simulink model "test_road"  (Simulink 7.6)
settings: Solver=ode3  StartTime=0.0  StopTime=10  FixedStep=.05  RelTol=1e-3
PostLoadFcn:
  | Threshold = 15;
  | MaxCluster = 25;
  | Num_Beams = 726;
  | Scaling = 1;
  | javaaddpath({'/'});
  | import ClusterMethodRoad.*;
  | DataCluster = ClusterMethodRoad(Threshold,MaxCluster,Scaling,8,0.33);
  | eml.extrinsic('evalin');
StartFcn:
  | md_scan(0);
StopFcn:
  | md_scan(2);
libraries: realtime_pacer_lib x1
settings Model: Creator=TCA  LastModifiedBy=Elliot
settings OptimizationCC: InitFltsAndDblsToZero=on
settings DebuggingCC: StrictBusMsg=Warning
settings SFSimCC: SimParseCustomCode=off

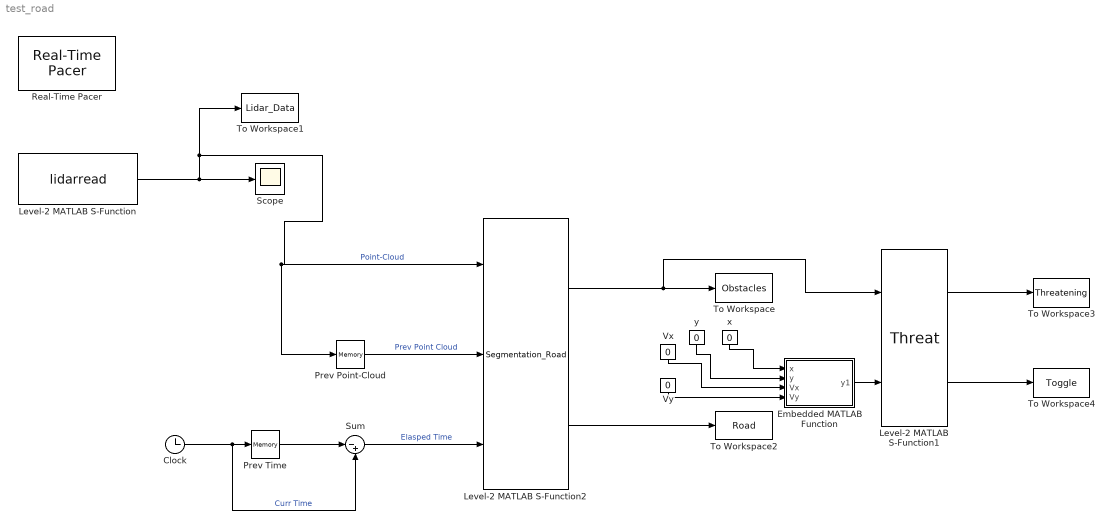
== system test_road ==
  Clock : Clock
      settings: Decimation=10
  Embedded MATLAB Function : Stateflow chart  TreatAsAtomicUnit=on
  Level-2 MATLAB S-Function : M-S-Function  FunctionName=lidarread
  Level-2 MATLAB S-Function1 : M-S-Function  FunctionName=Threat  Parameters=0.5,14,0.5
  Level-2 MATLAB S-Function2 : M-S-Function  FunctionName=Segmentation_Road
  Prev Point-Cloud : Memory
  Prev Time : Memory
  Real-Time Pacer : realtime_pacer_lib/Real-Time Pacer  simTimePerRealTime=1
  Scope : Scope
  Sum : Sum  Inputs=|-+
  To Workspace : ToWorkspace  VariableName=Obstacles  SampleTime=-1  SaveFormat=Structure
  To Workspace1 : ToWorkspace  VariableName=Lidar_Data  SampleTime=-1  SaveFormat=Structure With Time
  To Workspace2 : ToWorkspace  VariableName=Road  SampleTime=-1  SaveFormat=Structure
  To Workspace3 : ToWorkspace  VariableName=Threatening  SampleTime=-1  SaveFormat=Structure
  To Workspace4 : ToWorkspace  VariableName=Toggle  SampleTime=-1  SaveFormat=Array
  Vx : Constant  Value=0
  Vy : Constant  Value=0
  x : Constant  Value=0
  y : Constant  Value=0
  wires:
  Level-2 MATLAB S-Function/1 -> Scope/1, To Workspace1/1, Prev Point-Cloud/1, Level-2 MATLAB S-Function2/1  "Point-Cloud"
  Prev Point-Cloud/1 -> Level-2 MATLAB S-Function2/2  "Prev Point Cloud"
  Prev Time/1 -> Sum/1
  Sum/1 -> Level-2 MATLAB S-Function2/3  "Elasped Time"
  Clock/1 -> Prev Time/1, Sum/2  "Curr Time"
  Level-2 MATLAB S-Function2/1 -> To Workspace/1, Level-2 MATLAB S-Function1/1
  Level-2 MATLAB S-Function2/2 -> To Workspace2/1
  x/1 -> Embedded MATLAB Function/1(x)
  y/1 -> Embedded MATLAB Function/2(y)
  Vx/1 -> Embedded MATLAB Function/3(Vx)
  Vy/1 -> Embedded MATLAB Function/4(Vy)
  Embedded MATLAB Function/1(y1) -> Level-2 MATLAB S-Function1/2
  Level-2 MATLAB S-Function1/1 -> To Workspace3/1
  Level-2 MATLAB S-Function1/2 -> To Workspace4/1

== matlab function Embedded MATLAB Function ==
  data: x input double; y input double; Vx input double; Vy input double; y1 output double
function y1 = fcn(x,y,Vx,Vy)
%#eml
y1 = [x, y, Vx, Vy];
